simulink model "sajad_version_final_test"  (R2021b)
settings: Solver=VariableStepAuto  StartTime=0.0  StopTime=5  RelTol=1e-3
model workspace: external: MATLAB File D:\university\Semester 8\Intro to Robotics\Project\amali\Final_3\export second\Final_Assem_DataFile.m (data not in the file)
settings Model: Creator=admin  LastModifiedBy=admin

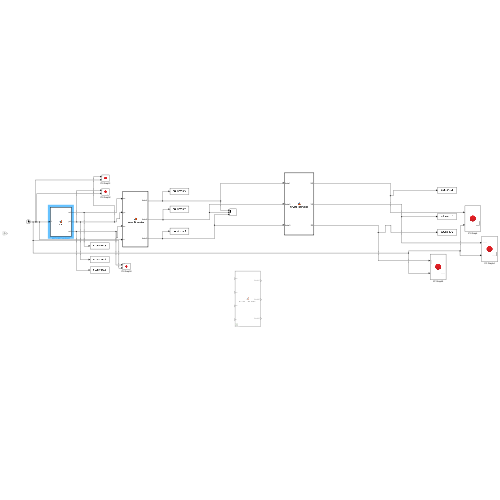
[thumbnail: Simulink's stored preview of the top-level diagram]
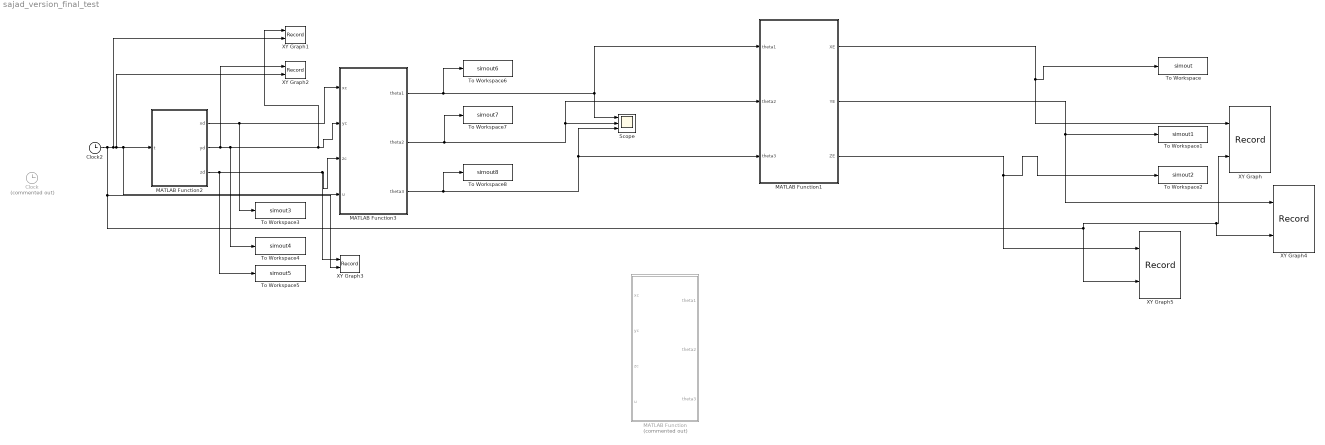
== system sajad_version_final_test ==
  Clock : Clock  Commented=on
      settings: Decimation=u
  Clock2 : Clock
      settings: Decimation=tt
  MATLAB Function : MATLAB Function  Commented=on  TreatAsAtomicUnit=on
  MATLAB Function1 : MATLAB Function  TreatAsAtomicUnit=on
  MATLAB Function2 : MATLAB Function  TreatAsAtomicUnit=on
  MATLAB Function3 : MATLAB Function  TreatAsAtomicUnit=on
  Scope : Scope  NumInputPorts=3
  To Workspace : ToWorkspace  VariableName=simout  SampleTime=-1
      settings: Save2DSignal=2-D array (concatenate along first dimension)
  To Workspace1 : ToWorkspace  VariableName=simout1  SampleTime=-1
      settings: Save2DSignal=2-D array (concatenate along first dimension)
  To Workspace2 : ToWorkspace  VariableName=simout2  SampleTime=-1
      settings: Save2DSignal=2-D array (concatenate along first dimension)
  To Workspace3 : ToWorkspace  VariableName=simout3  SampleTime=-1
      settings: Save2DSignal=2-D array (concatenate along first dimension)
  To Workspace4 : ToWorkspace  VariableName=simout4  SampleTime=-1
      settings: Save2DSignal=2-D array (concatenate along first dimension)
  To Workspace5 : ToWorkspace  VariableName=simout5  SampleTime=-1
      settings: Save2DSignal=2-D array (concatenate along first dimension)
  To Workspace6 : ToWorkspace  VariableName=simout6  SaveFormat=Timeseries  SampleTime=-1
      settings: Save2DSignal=2-D array (concatenate along first dimension)
  To Workspace7 : ToWorkspace  VariableName=simout7  SaveFormat=Timeseries  SampleTime=-1
  To Workspace8 : ToWorkspace  VariableName=simout8  SaveFormat=Timeseries  SampleTime=-1
  XY Graph : Record  FileSettingsInternal="{\"entries\":[{\"content\":{\"excelSettings\":{\"content\":{},\"type\":\"Streamout.ExcelSettings\"}},\"type\":\"Streamout.FileSettingStorage\",\"uuid\":\"7dac9fee-3216-47bc-8326-b7c482aa1b60\"}],\"packageUris\":[\"http://schema.mathworks.com/mf0/streamout_blocks/R2020a\"],\"version\":\"1.0\"}"  Layout=[1 1]  SignalsInternal="{\"entries\":[{\"content\":{\"signals\":[{\"content\":{\"blockPath\":[\"sajad_version_final_test/XY Graph\"],\"channel\":[],\"dimensions\":[1],\"domain\":\"sajad_version_final_test/XY Graph\",\"lineColor\":\"#fe330a\",\"plots\":[],\"port\":1,\"sid\":[\"\"],\"signalID\":2342,\"signalName\":\"MATLAB Function1:1\"},\"type\":\"RecordBlkView.Signal\",\"uuid\":\"7e77734a-cbdd-4bd9-980d-20a7776e7063\"},{\"content\":{\"blockPath\":[\"sajad_version_final_test/XY Graph\"],\"channel\":[],\"dimensions\":[1],\"domain\":\"sajad_version_final_test/XY Graph\",\"lineColor\":\"#22b573\",\"plots\":[],\"port\":2,\"sid\":[\"\"],\"signalID\":2346,\"signalName\":\"Clock2\"},\"type\":\"RecordBlkView.Signal\",\"uuid\":\"a98f09e5-3137-40a5-9068-44a075466e8d\"}]},\"type\":\"RecordBlkView.InputSignals\",\"uuid\":\"fb128054-4722-4e0c-a16e-3c5e6d06d634\"}],\"packageUris\":[\"http://schema.mathworks.com/mf0/streamout_blocks/R2020a\"],\"version\":\"1.0\"}"  VisualizationBindings="{\"xyplotplugin\":{\"info\":[{\"series\":[],\"subplotID\":1}]}}"  CompatibilityTag=XY
  XY Graph1 : Record  FileSettingsInternal="{\"entries\":[{\"content\":{\"excelSettings\":{\"content\":{},\"type\":\"Streamout.ExcelSettings\"}},\"type\":\"Streamout.FileSettingStorage\",\"uuid\":\"0c9f096c-6587-4c02-8025-8d0265fa37ff\"}],\"packageUris\":[\"http://schema.mathworks.com/mf0/streamout_blocks/R2020a\"],\"version\":\"1.0\"}"  Layout=[1 1]  SignalsInternal="{\"entries\":[{\"content\":{\"signals\":[{\"content\":{\"blockPath\":[\"sajad_version_final_test/XY Graph1\"],\"channel\":[],\"dimensions\":[1],\"domain\":\"sajad_version_final_test/XY Graph1\",\"lineColor\":\"#0072bd\",\"plots\":[],\"port\":1,\"sid\":[\"\"],\"signalID\":2350,\"signalName\":\"MATLAB Function2:2\"},\"type\":\"RecordBlkView.Signal\",\"uuid\":\"bb97a7f4-1a47-4c81-b4f8-75564929aa4a\"},{\"content\":{\"blockPath\":[\"sajad_version_final_test/XY Graph1\"],\"channel\":[],\"dimensions\":[1],\"domain\":\"sajad_version_final_test/XY Graph1\",\"lineColor\":\"#d95319\",\"plots\":[],\"port\":2,\"sid\":[\"\"],\"signalID\":2354,\"signalName\":\"Clock2\"},\"type\":\"RecordBlkView.Signal\",\"uuid\":\"832467d8-e53c-4869-bfe4-3217613d7668\"}]},\"type\":\"RecordBlkView.InputSignals\",\"uuid\":\"eeb17bda-6131-40b2-b8da-3e48eef50d1a\"}],\"packageUris\":[\"http://schema.mathworks.com/mf0/streamout_blocks/R2020a\"],\"version\":\"1.0\"}"  VisualizationBindings="{\"xyplotplugin\":{\"info\":[{\"series\":[],\"subplotID\":1}]}}"  CompatibilityTag=XY
  XY Graph2 : Record  FileSettingsInternal="{\"entries\":[{\"content\":{\"excelSettings\":{\"content\":{},\"type\":\"Streamout.ExcelSettings\"}},\"type\":\"Streamout.FileSettingStorage\",\"uuid\":\"5b88a4d1-b4ee-49b2-8a74-785bd9d41aac\"}],\"packageUris\":[\"http://schema.mathworks.com/mf0/streamout_blocks/R2020a\"],\"version\":\"1.0\"}"  Layout=[1 1]  SignalsInternal="{\"entries\":[{\"content\":{\"signals\":[{\"content\":{\"blockPath\":[\"sajad_version_final_test/XY Graph2\"],\"channel\":[],\"dimensions\":[1],\"domain\":\"sajad_version_final_test/XY Graph2\",\"lineColor\":\"#edb120\",\"plots\":[],\"port\":1,\"sid\":[\"\"],\"signalID\":2358,\"signalName\":\"MATLAB Function2:2\"},\"type\":\"RecordBlkView.Signal\",\"uuid\":\"435b0cea-1e1e-4639-9588-c5e491f32352\"},{\"content\":{\"blockPath\":[\"sajad_version_final_test/XY Graph2\"],\"channel\":[],\"dimensions\":[1],\"domain\":\"sajad_version_final_test/XY Graph2\",\"lineColor\":\"#7e2f8e\",\"plots\":[],\"port\":2,\"sid\":[\"\"],\"signalID\":2362,\"signalName\":\"Clock2\"},\"type\":\"RecordBlkView.Signal\",\"uuid\":\"f0a0417b-3546-486b-89cb-6095c0a38fae\"}]},\"type\":\"RecordBlkView.InputSignals\",\"uuid\":\"ca8e09ad-31b6-4162-a679-00a45b8bb8d7\"}],\"packageUris\":[\"http://schema.mathworks.com/mf0/streamout_blocks/R2020a\"],\"version\":\"1.0\"}"  VisualizationBindings="{\"xyplotplugin\":{\"info\":[{\"series\":[],\"subplotID\":1}]}}"  CompatibilityTag=XY
  XY Graph3 : Record  FileSettingsInternal="{\"entries\":[{\"content\":{\"excelSettings\":{\"content\":{},\"type\":\"Streamout.ExcelSettings\"}},\"type\":\"Streamout.FileSettingStorage\",\"uuid\":\"d800a2e1-31d1-451a-8e4d-dfe295e0a662\"}],\"packageUris\":[\"http://schema.mathworks.com/mf0/streamout_blocks/R2020a\"],\"version\":\"1.0\"}"  Layout=[1 1]  SignalsInternal="{\"entries\":[{\"content\":{\"signals\":[{\"content\":{\"blockPath\":[\"sajad_version_final_test/XY Graph3\"],\"channel\":[],\"dimensions\":[1],\"domain\":\"sajad_version_final_test/XY Graph3\",\"lineColor\":\"#77ac30\",\"plots\":[],\"port\":1,\"sid\":[\"\"],\"signalID\":2366,\"signalName\":\"MATLAB Function2:3\"},\"type\":\"RecordBlkView.Signal\",\"uuid\":\"5064f439-457d-4a66-a3d4-a6fa77be6661\"},{\"content\":{\"blockPath\":[\"sajad_version_final_test/XY Graph3\"],\"channel\":[],\"dimensions\":[1],\"domain\":\"sajad_version_final_test/XY Graph3\",\"lineColor\":\"#4dbeee\",\"plots\":[],\"port\":2,\"sid\":[\"\"],\"signalID\":2370,\"signalName\":\"Clock2\"},\"type\":\"RecordBlkView.Signal\",\"uuid\":\"8fcf9e1c-e45d-4b55-a294-314482cd506c\"}]},\"type\":\"RecordBlkView.InputSignals\",\"uuid\":\"3c884bfb-25fa-4797-9fd8-5fb6020b3edc\"}],\"packageUris\":[\"http://schema.mathworks.com/mf0/streamout_blocks/R2020a\"],\"version\":\"1.0\"}"  VisualizationBindings="{\"xyplotplugin\":{\"info\":[{\"series\":[],\"subplotID\":1}]}}"  CompatibilityTag=XY
  XY Graph4 : Record  FileSettingsInternal="{\"entries\":[{\"content\":{\"excelSettings\":{\"content\":{},\"type\":\"Streamout.ExcelSettings\"}},\"type\":\"Streamout.FileSettingStorage\",\"uuid\":\"49b56f05-c569-49de-ac35-0a2ee0e80fec\"}],\"packageUris\":[\"http://schema.mathworks.com/mf0/streamout_blocks/R2020a\"],\"version\":\"1.0\"}"  Layout=[1 1]  SignalsInternal="{\"entries\":[{\"content\":{\"signals\":[{\"content\":{\"blockPath\":[\"sajad_version_final_test/XY Graph4\"],\"channel\":[],\"dimensions\":[1],\"domain\":\"sajad_version_final_test/XY Graph4\",\"lineColor\":\"#a2142f\",\"plots\":[],\"port\":1,\"sid\":[\"\"],\"signalID\":2374,\"signalName\":\"MATLAB Function1:2\"},\"type\":\"RecordBlkView.Signal\",\"uuid\":\"a183b6bc-f9d8-4346-a4b3-d44085ed926f\"},{\"content\":{\"blockPath\":[\"sajad_version_final_test/XY Graph4\"],\"channel\":[],\"dimensions\":[1],\"domain\":\"sajad_version_final_test/XY Graph4\",\"lineColor\":\"#139fff\",\"plots\":[],\"port\":2,\"sid\":[\"\"],\"signalID\":2378,\"signalName\":\"Clock2\"},\"type\":\"RecordBlkView.Signal\",\"uuid\":\"b56a4c62-fc97-43fa-9d81-33f8aa9fbe6e\"}]},\"type\":\"RecordBlkView.InputSignals\",\"uuid\":\"e0e07585-7efb-4fe5-9e29-911b882203ec\"}],\"packageUris\":[\"http://schema.mathworks.com/mf0/streamout_blocks/R2020a\"],\"version\":\"1.0\"}"  VisualizationBindings="{\"xyplotplugin\":{\"info\":[{\"series\":[],\"subplotID\":1}]}}"  CompatibilityTag=XY
  XY Graph5 : Record  FileSettingsInternal="{\"entries\":[{\"content\":{\"excelSettings\":{\"content\":{},\"type\":\"Streamout.ExcelSettings\"}},\"type\":\"Streamout.FileSettingStorage\",\"uuid\":\"00d11316-e04b-49dd-89ee-f96781c43d62\"}],\"packageUris\":[\"http://schema.mathworks.com/mf0/streamout_blocks/R2020a\"],\"version\":\"1.0\"}"  Layout=[1 1]  SignalsInternal="{\"entries\":[{\"content\":{\"signals\":[{\"content\":{\"blockPath\":[\"sajad_version_final_test/XY Graph5\"],\"channel\":[],\"dimensions\":[1],\"domain\":\"sajad_version_final_test/XY Graph5\",\"lineColor\":\"#ff6929\",\"plots\":[],\"port\":1,\"sid\":[\"\"],\"signalID\":2382,\"signalName\":\"MATLAB Function1:3\"},\"type\":\"RecordBlkView.Signal\",\"uuid\":\"0034d8d5-0289-4312-b49e-fd87ebd550f6\"},{\"content\":{\"blockPath\":[\"sajad_version_final_test/XY Graph5\"],\"channel\":[],\"dimensions\":[1],\"domain\":\"sajad_version_final_test/XY Graph5\",\"lineColor\":\"#b746ff\",\"plots\":[],\"port\":2,\"sid\":[\"\"],\"signalID\":2386,\"signalName\":\"Clock2\"},\"type\":\"RecordBlkView.Signal\",\"uuid\":\"0a955c30-cdcc-496b-a44d-512d2614c767\"}]},\"type\":\"RecordBlkView.InputSignals\",\"uuid\":\"54e2fabd-cf25-418a-897a-2b9b0cf1ff05\"}],\"packageUris\":[\"http://schema.mathworks.com/mf0/streamout_blocks/R2020a\"],\"version\":\"1.0\"}"  VisualizationBindings="{\"xyplotplugin\":{\"info\":[{\"series\":[],\"subplotID\":1}]}}"  CompatibilityTag=XY
  wires:
  MATLAB Function2/1(xd) -> MATLAB Function3/1(xc), To Workspace3/1
  MATLAB Function2/2(yd) -> XY Graph2/1, To Workspace4/1, MATLAB Function3/2(yc), XY Graph1/1
  MATLAB Function2/3(zd) -> To Workspace5/1, MATLAB Function3/3(zc), XY Graph3/1
  MATLAB Function1/1(XE) -> XY Graph/1, To Workspace/1
  MATLAB Function1/2(YE) -> XY Graph4/1, To Workspace1/1
  MATLAB Function1/3(ZE) -> XY Graph5/1, To Workspace2/1
  Clock2/1 -> XY Graph3/2, XY Graph4/2, XY Graph/2, XY Graph5/2, XY Graph1/2, XY Graph2/2, MATLAB Function3/4(u), MATLAB Function2/1(t)
  MATLAB Function3/1(theta1) -> To Workspace6/1, Scope/1, MATLAB Function1/1(theta1)
  MATLAB Function3/2(theta2) -> To Workspace7/1, Scope/2, MATLAB Function1/2(theta2)
  MATLAB Function3/3(theta3) -> To Workspace8/1, Scope/3, MATLAB Function1/3(theta3)

== matlab function sajad_version_final_test/MATLAB Function1 ==
  data: theta1 input; XE output; theta2 input; theta3 input; YE output; ZE output
function [XE,YE,ZE]= forward_kinematics(theta1,theta2, theta3)
% 
% 
% xa= 0.224*cos(theta1)*sin(theta2) - 0.06821*cos(theta1) + 0.1*cos(theta1)*cos(theta2)*sin(theta3) + 0.1*cos(theta1)*cos(theta3)*sin(theta2);
% ya= 0.224*cos(theta1)*sin(theta2) - 0.06821*cos(theta1) + 0.1*cos(theta1)*cos(theta2)*sin(theta3) + 0.1*cos(theta1)*cos(theta3)*sin(theta2);
% za= 0.1*cos(theta2 + theta3) + 0.224*cos(theta2) + 0.178;

%a
a1=0;  %%% actualy a0
a2=-0.0165; %%% actualy a1
a3=0.217;   %%% L2   actualy a2
a4=0;     %%   actualy a3
%alpha
alphab1=  0;
alphab2= -pi/2;
alphab3=  0;
alphab4= -pi/2;
% d
d1 = 0.2867;
d2 = 0;
d3 = 0;
d4 = 0.1;  %%% L3
%theta
% theta2 = 0;
% theta3 = 0;
 theta4 =0;
T1=[cos(theta1) -sin(theta1) 0 a1;
   sin(theta1)*cos(alphab1) cos(theta1)*cos(alphab1) -sin(alphab1) -sin(alphab1)*d1;
   sin(theta1)*sin(alphab1) cos(theta1)*sin(alphab1) cos(alphab1) cos(alphab1)*d1;
   0 0 0 1];
T2=[cos(theta2) -sin(theta2) 0 a2;
   sin(theta2)*cos(alphab2) cos(theta2)*cos(alphab2) -sin(alphab2) -sin(alphab2)*d2;
   sin(theta2)*sin(alphab2) cos(theta2)*sin(alphab2) cos(alphab2) cos(alphab2)*d2;
   0 0 0 1];
T3=[cos(theta3) -sin(theta3) 0 a3;
   sin(theta3)*cos(alphab3) cos(theta3)*cos(alphab3) -sin(alphab3) -sin(alphab3)*d3;
   sin(theta3)*sin(alphab3) cos(theta3)*sin(alphab3) cos(alphab3) cos(alphab3)*d3;
   0 0 0 1];
 T4=[cos(theta4) -sin(theta4) 0 a4;
    sin(theta4)*cos(alphab4) cos(theta4)*cos(alphab4) -sin(alphab4) -sin(alphab4)*d4;
   sin(theta4)*sin(alphab4) cos(theta4)*sin(alphab4) cos(alphab4) cos(alphab4)*d4;
    0 0 0 1];
Ttotal = T1*T2*T3*T4;
XE = Ttotal(1,4);
YE = Ttotal(2,4);
ZE = Ttotal(3,4);

== matlab function sajad_version_final_test/MATLAB Function ==
  data: xc input; theta1 output; yc input; zc input; theta2 output; theta3 output; u input
function [theta1,theta2,theta3]= inverse_kinematics(xc,yc,zc,u)
theta1 = atan2(yc,xc)

xprim = (xc /cos(theta1))+ 0.0682;
yprim = (yc /sin(theta1))+0.0682;
zprim = zc - 0.178;
c_3 = (yprim^2+zprim^2-0.06)/(0.0449);
s_3 =(1-(1/2)*c_3^2);
theta3 = atan2(s_3,c_3)

c_2=((0.224*cos(theta1)+0.1*cos(theta3)*cos(theta1))*(zc-0.178))-(0.1*cos(theta3)*(xc+0.0682));
s_2=((xc+0.0682)*(0.1*sin(theta3)+0.224))-(zc-0.178)*(0.1*sin(theta3)*cos(theta1));
theta2 = atan2(s_2,c_2)
% d= 0.0165;
% d1= 0.196;
% a2= 0.217;
% a3=0.1;
% phi= atan2(xc,yc);
% r=sqrt(xc^2+yc^2);
% alpha= atan2(sqrt(r^2-d^2),d);
% theta1= phi- alpha
% s= zc-d1;
% rprim= sqrt(xc^2+yc^2-d^2);
% D= (rprim^2+s^2 - a2^2 - a3^2)/(2*a2*a3);
% if(u<5)
% theta3= atan2(D,sqrt(abs(1-D^2)))
% theta2=atan2(rprim,s)- atan2(a2 + a3*cos(theta3),a3*sin(theta3))
% else
% theta3= atan2(D,-sqrt(abs(1-D^2)));
% theta2=atan2(rprim,s)- atan2(a2 + a3*cos(theta3),a3*sin(theta3))
% end

== matlab function sajad_version_final_test/MATLAB Function2 ==
  data: t input; xd output; yd output; zd output
function [xd,yd,zd]=DT(t)

% xd= 0.2 - 0.2*sin((2*pi/5)*u + pi/2);
% yd= 0.3; %-1 - 0.5*cos((2*pi/5)*u + pi/2);
% zd= -0.5 - 0.5*cos((2*pi/5)*u + pi/2);
% if(t<5)
x0=0.09;  %0.15
y0=0.09;  %0.15
z0=0.09; %1
x1=0.05; %-0.05
y1=0.05;  %0.05
z1=0.05; %2
s=t/5;
xd=x0+(x1-x0)*s; 
yd=y0+(y1-y0)*s;
zd=z0+(z1-z0)*s;
% else
% x0=0.05;
% y0=-0.05; %0.1
% z0=0.4;
% x1=0.1;
% y1=0.1;
% z1=0.15;
% s=(t-5)/5;
% xd=x0+(x1-x0)*s; 
% yd=y0+(y1-y0)*s;
% zd=z0+(z1-z0)*s;
% % v = (qi-qf)/(tb-tf)
end

== matlab function sajad_version_final_test/MATLAB Function3 ==
  data: xc input; theta1 output; yc input; zc input; theta2 output; theta3 output; u input
function [theta1,theta2,theta3]= inverse_kinematics(xc,yc,zc,u)
% d= 0.0165;
% d1= 0.196;
% d1 = 0.2867;
% a2=-0.0165; %%% actualy a1
% a3=0.217;   %%% L2   actualy a2
% a2= 0.217;
% a3=0.1;
% phi= atan2(xc,yc);
% r=sqrt(xc^2+yc^2);
% alpha= atan2(sqrt(r^2-d^2),d);
% theta1= phi- alpha;
% s= zc-d1;
% rprim= sqrt(xc^2+yc^2-d^2);
% D= (rprim^2+s^2 - a2^2 - a3^2)/(2*a2*a3);
% % if(u<5)
% theta3= atan2(D,sqrt(abs(1-D^2)));
% theta2=atan2(rprim,s)- atan2(a2 + a3*cos(theta3),a3*sin(theta3));
% else
% theta3= atan2(D,-sqrt(abs(1-D^2)));
% theta2=atan2(rprim,s)- atan2(a2 + a3*cos(theta3),a3*sin(theta3))

theta1=atan2(yc,xc)
xprim=(xc/cos(theta1))+0.0165;
yprim=(yc/sin(theta1))+0.0165;
zprim=-zc+0.2867;
st3=(0.217^2 + 0.1^2 - zprim^2 - yprim^2)/(0.217*2*0.1);
ct3=sqrt(1-st3^2);
theta3=atan2(st3,ct3)
denom=((0.217*cos(theta1)-0.1*sin(theta3)*cos(theta1))*(-0.1*sin(theta1)*cos(theta3)))-(0.217*sin(theta1)-0.1*sin(theta3)*sin(theta1))*(-0.1*cos(theta3)*cos(theta1));
numc= ((xc+0.0165*cos(theta1))*(-0.1*sin(theta1)*cos(theta3))) - (yc+0.0165*sin(theta1))*(-0.1*cos(theta3)*cos(theta1));
ct2=numc/denom;
nums= ((0.217*cos(theta1)-0.1*sin(theta3)*cos(theta1))*(yc+0.0165*sin(theta1))) - (0.217*sin(theta1)-0.1*sin(theta3)*sin(theta1))*(xc+0.0165*cos(theta1));
st2=nums/denom;
% st2=sqrt(1-ct2^2);
theta2=atan2(st2,ct2)

 end
